simulink model "DDCU_wxt_v02_forA_OpenLoop"  (R2014a)
settings: Solver=FixedStepDiscrete  StartTime=0.0  StopTime=16  FixedStep=0.05  RelTol=1e-3
InitFcn:
  | Veh_Par_wxt
values from neighbouring files (symbols this model uses):
  ag_thr = 0.4*g    (= 3.924)    [Veh_Par_wxt.m]
  B = 2.25    [Veh_Par_wxt.m]
  bra_pre_em = 12    [Veh_Par_wxt.m]
  bra_pre_gz2 = 12/3    (= 4)    [Veh_Par_wxt.m]
  bra_pre_gz34 = 12/3    (= 4)    [Veh_Par_wxt.m]
  bra_pre_yd = 12/2    (= 6)    [Veh_Par_wxt.m]
  brakepre_dem_data = [0 1 2 3 4 5 6 7 8 9 10 11 12]    [Veh_Par_wxt.m]
  brakeTrq_dem_data = [0 218.198 436.396 654.594 872.792 1090.99 1309.188 1527.386 1745.584 1963.782 2181.98 2400.178 2618.376]    [Veh_Par_wxt.m]
  bratrq_max = 4*2618.376    (= 10473.504)    [Veh_Par_wxt.m]
  eff_tran = 0.75    [Veh_Par_wxt.m]
  G = Mass*g    (= 36297)    [Veh_Par_wxt.m]
  kd1 = 1    [Veh_Par_wxt.m]
  kd2 = 1    [Veh_Par_wxt.m]
  kd3 = 1    [Veh_Par_wxt.m]
  ki1 = 1    [Veh_Par_wxt.m]
  ki2 = 1    [Veh_Par_wxt.m]
  ki3 = 1    [Veh_Par_wxt.m]
  kp1 = 1    [Veh_Par_wxt.m]
  kp2 = 1    [Veh_Par_wxt.m]
  kp3 = 1    [Veh_Par_wxt.m]
  L = 3.12    [Veh_Par_wxt.m]
  premax = 12    [Veh_Par_wxt.m]
  Radius = 0.20    (= 0.2)    [Veh_Par_wxt.m]
  s_opt_yi_add = 0.05    [Veh_Par_wxt.m]
  s_opt_zhuan_add = 0.05    [Veh_Par_wxt.m]
  spd_map_mot = [0 100 200 300 360 400 500 600 700 800 900]*tras_ratio    [Veh_Par_wxt.m]
  spdmax = 900*tras_ratio    (= 5580)    [Veh_Par_wxt.m]
  speed_thr_park = 5/3.6/Radius*30/pi    (= 66.3145596216)    [Veh_Par_wxt.m]
  tras_ratio = 6.2    [Veh_Par_wxt.m]
  trq_map_mot = [1200 1200 1200 1200 1200 1080 864 720 617 540 480]/tras_ratio    [Veh_Par_wxt.m]
  trqmax = 80    [Veh_Par_wxt.m]
  v_thr1_b = 5    [Veh_Par_wxt.m]
  v_thr2_b = 20    [Veh_Par_wxt.m]
  v_thr_park = 5    [Veh_Par_wxt.m]
undefined symbols (not defined in the file or in its folder): DiscIntNeverNeededParam, sigbuilder_block
libraries: simulink x169, ec5744lib x9
(part 4 of 13)

== system DDCU_wxt_v02_forA_OpenLoop/OutputSignalProcess/VCU_MCU1_replace/M2Mode ==
  M2Mode : Inport
  Constant{1..4,6..8} (7 alike) : Constant  Value=0  OutDataTypeStr=uint8
  M2ModeRon : Rounding  Operator=round
  M2Mode_1sat : Saturate  UpperLimit=3  LowerLimit=0
  M2Mode_Convert : DataTypeConversion  OutDataTypeStr=uint8
  M2Mode_Convert1 : DataTypeConversion  OutDataTypeStr=uint32
  M2Mode_D : Product  Inputs=*/
  M2Mode_F : Constant  OutDataTypeStr=single
  M2Mode_L : simulink/Logic and Bit Operations/Bitwise Operator  logicop=AND  UseBitMask=on  BitMask=3  BitMaskRealWorld=Stored Integer
  M2Mode_O : Constant  Value=0  OutDataTypeStr=single
  M2Mode_S : ArithShift
  M2Mode_sat : Saturate  UpperLimit=3  LowerLimit=0
  M2Mode_st : Sum  Inputs=+-
  output1 : Outport
  output2 : Outport  Port=2
  output3 : Outport  Port=3
  output4 : Outport  Port=4
  output5 : Outport  Port=5
  output6 : Outport  Port=6
  output7 : Outport  Port=7
  output8 : Outport  Port=8
  wires:
  M2Mode/1 -> M2Mode_sat/1
  M2Mode_sat/1 -> M2Mode_st/1
  M2Mode_O/1 -> M2Mode_st/2
  M2Mode_st/1 -> M2Mode_D/1
  M2Mode_F/1 -> M2Mode_D/2
  M2Mode_D/1 -> M2ModeRon/1
  M2ModeRon/1 -> M2Mode_S/1
  M2Mode_S/1 -> M2Mode_1sat/1
  M2Mode_1sat/1 -> M2Mode_Convert1/1
  M2Mode_Convert1/1 -> M2Mode_L/1
  M2Mode_L/1 -> M2Mode_Convert/1
  M2Mode_Convert/1 -> output5/1
  Constant1/1 -> output1/1
  Constant2/1 -> output2/1
  Constant3/1 -> output3/1
  Constant4/1 -> output4/1
  Constant6/1 -> output6/1
  Constant7/1 -> output7/1
  Constant8/1 -> output8/1

== system DDCU_wxt_v02_forA_OpenLoop/OutputSignalProcess/VCU_MCU1_replace/M2SpeedLimit ==
  M2SpeedLimit : Inport
  Constant{1..6} (6 alike) : Constant  Value=0  OutDataTypeStr=uint8
  M2SpeedLimitBitCov : DataTypeConversion  OutDataTypeStr=uint8
  M2SpeedLimitCOV : DataTypeConversion  OutDataTypeStr=uint8
  M2SpeedLimitRon : Rounding  Operator=round
  M2SpeedLimit_1sat : Saturate  UpperLimit=4095  LowerLimit=0
  M2SpeedLimit_And : simulink/Logic and Bit Operations/Bitwise Operator  logicop=AND  UseBitMask=off  NumInputPorts=2  BitMask=bin2dec('11011001')  BitMaskRealWorld=Stored Integer
  M2SpeedLimit_And_C : Constant  Value=255  OutDataTypeStr=uint32
  M2SpeedLimit_Convert : DataTypeConversion  OutDataTypeStr=uint32
  M2SpeedLimit_D : Product  Inputs=*/
  M2SpeedLimit_D1 : Product  Inputs=*/
  M2SpeedLimit_F : Constant  Value=5  OutDataTypeStr=single
  M2SpeedLimit_L : simulink/Logic and Bit Operations/Bitwise Operator  logicop=AND  UseBitMask=on  BitMask=4095  BitMaskRealWorld=Stored Integer
  M2SpeedLimit_O : Constant  Value=0  OutDataTypeStr=single
  M2SpeedLimit_S : ArithShift
  M2SpeedLimit_sat : Saturate  UpperLimit=20475  LowerLimit=0
  M2SpeedLimit_st : Sum  Inputs=+-
  M2SpeedLimitoutput8_C : Constant  Value=256
  output1 : Outport
  output2 : Outport  Port=2
  output3 : Outport  Port=3
  output4 : Outport  Port=4
  output5 : Outport  Port=5
  output6 : Outport  Port=6
  output7 : Outport  Port=7
  output8 : Outport  Port=8
  wires:
  M2SpeedLimit/1 -> M2SpeedLimit_sat/1
  M2SpeedLimit_sat/1 -> M2SpeedLimit_st/1
  M2SpeedLimit_O/1 -> M2SpeedLimit_st/2
  M2SpeedLimit_st/1 -> M2SpeedLimit_D/1
  M2SpeedLimit_F/1 -> M2SpeedLimit_D/2
  M2SpeedLimit_D/1 -> M2SpeedLimitRon/1
  M2SpeedLimitRon/1 -> M2SpeedLimit_S/1
  M2SpeedLimit_S/1 -> M2SpeedLimit_1sat/1
  M2SpeedLimit_1sat/1 -> M2SpeedLimit_Convert/1
  M2SpeedLimit_Convert/1 -> M2SpeedLimit_L/1
  M2SpeedLimit_L/1 -> M2SpeedLimit_D1/1, M2SpeedLimit_And/1
  M2SpeedLimitoutput8_C/1 -> M2SpeedLimit_D1/2
  M2SpeedLimit_D1/1 -> M2SpeedLimitCOV/1
  M2SpeedLimitCOV/1 -> output8/1
  M2SpeedLimit_And_C/1 -> M2SpeedLimit_And/2
  M2SpeedLimit_And/1 -> M2SpeedLimitBitCov/1
  M2SpeedLimitBitCov/1 -> output7/1
  Constant1/1 -> output1/1
  Constant2/1 -> output2/1
  Constant3/1 -> output3/1
  Constant4/1 -> output4/1
  Constant5/1 -> output5/1
  Constant6/1 -> output6/1

== system DDCU_wxt_v02_forA_OpenLoop/OutputSignalProcess/VCU_MCU1_replace/M2SpeedSet ==
  M2SpeedSet : Inport
  Constant{1..4,7..8} (6 alike) : Constant  Value=0  OutDataTypeStr=uint8
  M2SpeedSetBitCov : DataTypeConversion  OutDataTypeStr=uint8
  M2SpeedSetCOV : DataTypeConversion  OutDataTypeStr=uint8
  M2SpeedSetRon : Rounding  Operator=round
  M2SpeedSet_1sat : Saturate  UpperLimit=65520  LowerLimit=0
  M2SpeedSet_And : simulink/Logic and Bit Operations/Bitwise Operator  logicop=AND  UseBitMask=off  NumInputPorts=2  BitMask=bin2dec('11011001')  BitMaskRealWorld=Stored Integer
  M2SpeedSet_And_C : Constant  Value=255  OutDataTypeStr=uint32
  M2SpeedSet_Convert : DataTypeConversion  OutDataTypeStr=uint32
  M2SpeedSet_D : Product  Inputs=*/
  M2SpeedSet_D1 : Product  Inputs=*/
  M2SpeedSet_F : Constant  Value=5  OutDataTypeStr=single
  M2SpeedSet_L : simulink/Logic and Bit Operations/Bitwise Operator  logicop=AND  UseBitMask=on  BitMask=65520  BitMaskRealWorld=Stored Integer
  M2SpeedSet_O : Constant  Value=-5000  OutDataTypeStr=single
  M2SpeedSet_S : ArithShift  BitShiftNumber=-4
  M2SpeedSet_sat : Saturate  UpperLimit=15475  LowerLimit=-5000
  M2SpeedSet_st : Sum  Inputs=+-
  M2SpeedSetoutput6_C : Constant  Value=256
  output1 : Outport
  output2 : Outport  Port=2
  output3 : Outport  Port=3
  output4 : Outport  Port=4
  output5 : Outport  Port=5
  output6 : Outport  Port=6
  output7 : Outport  Port=7
  output8 : Outport  Port=8
  wires:
  M2SpeedSet/1 -> M2SpeedSet_sat/1
  M2SpeedSet_sat/1 -> M2SpeedSet_st/1
  M2SpeedSet_O/1 -> M2SpeedSet_st/2
  M2SpeedSet_st/1 -> M2SpeedSet_D/1
  M2SpeedSet_F/1 -> M2SpeedSet_D/2
  M2SpeedSet_D/1 -> M2SpeedSetRon/1
  M2SpeedSetRon/1 -> M2SpeedSet_S/1
  M2SpeedSet_S/1 -> M2SpeedSet_1sat/1
  M2SpeedSet_1sat/1 -> M2SpeedSet_Convert/1
  M2SpeedSet_Convert/1 -> M2SpeedSet_L/1
  M2SpeedSet_L/1 -> M2SpeedSet_D1/1, M2SpeedSet_And/1
  M2SpeedSetoutput6_C/1 -> M2SpeedSet_D1/2
  M2SpeedSet_D1/1 -> M2SpeedSetCOV/1
  M2SpeedSetCOV/1 -> output6/1
  M2SpeedSet_And_C/1 -> M2SpeedSet_And/2
  M2SpeedSet_And/1 -> M2SpeedSetBitCov/1
  M2SpeedSetBitCov/1 -> output5/1
  Constant1/1 -> output1/1
  Constant2/1 -> output2/1
  Constant3/1 -> output3/1
  Constant4/1 -> output4/1
  Constant7/1 -> output7/1
  Constant8/1 -> output8/1

== system DDCU_wxt_v02_forA_OpenLoop/OutputSignalProcess/VCU_MCU1_replace/MCU1HeartBeat ==
  MCU1HeartBeat : Inport
  Constant{1..7} (7 alike) : Constant  Value=0  OutDataTypeStr=uint8
  MCU1HeartBeatRon : Rounding  Operator=round
  MCU1HeartBeat_1sat : Saturate  UpperLimit=240  LowerLimit=0
  MCU1HeartBeat_Convert : DataTypeConversion  OutDataTypeStr=uint8
  MCU1HeartBeat_Convert1 : DataTypeConversion  OutDataTypeStr=uint32
  MCU1HeartBeat_D : Product  Inputs=*/
  MCU1HeartBeat_F : Constant  OutDataTypeStr=single
  MCU1HeartBeat_L : simulink/Logic and Bit Operations/Bitwise Operator  logicop=AND  UseBitMask=on  BitMask=240  BitMaskRealWorld=Stored Integer
  MCU1HeartBeat_O : Constant  Value=0  OutDataTypeStr=single
  MCU1HeartBeat_S : ArithShift  BitShiftNumber=-4
  MCU1HeartBeat_sat : Saturate  UpperLimit=15  LowerLimit=0
  MCU1HeartBeat_st : Sum  Inputs=+-
  output1 : Outport
  output2 : Outport  Port=2
  output3 : Outport  Port=3
  output4 : Outport  Port=4
  output5 : Outport  Port=5
  output6 : Outport  Port=6
  output7 : Outport  Port=7
  output8 : Outport  Port=8
  wires:
  MCU1HeartBeat/1 -> MCU1HeartBeat_sat/1
  MCU1HeartBeat_sat/1 -> MCU1HeartBeat_st/1
  MCU1HeartBeat_O/1 -> MCU1HeartBeat_st/2
  MCU1HeartBeat_st/1 -> MCU1HeartBeat_D/1
  MCU1HeartBeat_F/1 -> MCU1HeartBeat_D/2
  MCU1HeartBeat_D/1 -> MCU1HeartBeatRon/1
  MCU1HeartBeatRon/1 -> MCU1HeartBeat_S/1
  MCU1HeartBeat_S/1 -> MCU1HeartBeat_1sat/1
  MCU1HeartBeat_1sat/1 -> MCU1HeartBeat_Convert1/1
  MCU1HeartBeat_Convert1/1 -> MCU1HeartBeat_L/1
  MCU1HeartBeat_L/1 -> MCU1HeartBeat_Convert/1
  MCU1HeartBeat_Convert/1 -> output8/1
  Constant1/1 -> output1/1
  Constant2/1 -> output2/1
  Constant3/1 -> output3/1
  Constant4/1 -> output4/1
  Constant5/1 -> output5/1
  Constant6/1 -> output6/1
  Constant7/1 -> output7/1

== system DDCU_wxt_v02_forA_OpenLoop/OutputSignalProcess/VCU_MCU2/M3Drive ==
  M3Drive : Inport
  Constant{2..8} (7 alike) : Constant  Value=0  OutDataTypeStr=uint8
  M3DriveRon : Rounding  Operator=round
  M3Drive_1sat : Saturate  UpperLimit=48  LowerLimit=0
  M3Drive_Convert : DataTypeConversion  OutDataTypeStr=uint8
  M3Drive_Convert1 : DataTypeConversion  OutDataTypeStr=uint32
  M3Drive_D : Product  Inputs=*/
  M3Drive_F : Constant  OutDataTypeStr=single
  M3Drive_L : simulink/Logic and Bit Operations/Bitwise Operator  logicop=AND  UseBitMask=on  BitMask=48  BitMaskRealWorld=Stored Integer
  M3Drive_O : Constant  Value=0  OutDataTypeStr=single
  M3Drive_S : ArithShift  BitShiftNumber=-4
  M3Drive_sat : Saturate  UpperLimit=3  LowerLimit=0
  M3Drive_st : Sum  Inputs=+-
  output1 : Outport
  output2 : Outport  Port=2
  output3 : Outport  Port=3
  output4 : Outport  Port=4
  output5 : Outport  Port=5
  output6 : Outport  Port=6
  output7 : Outport  Port=7
  output8 : Outport  Port=8
  wires:
  M3Drive/1 -> M3Drive_sat/1
  M3Drive_sat/1 -> M3Drive_st/1
  M3Drive_O/1 -> M3Drive_st/2
  M3Drive_st/1 -> M3Drive_D/1
  M3Drive_F/1 -> M3Drive_D/2
  M3Drive_D/1 -> M3DriveRon/1
  M3DriveRon/1 -> M3Drive_S/1
  M3Drive_S/1 -> M3Drive_1sat/1
  M3Drive_1sat/1 -> M3Drive_Convert1/1
  M3Drive_Convert1/1 -> M3Drive_L/1
  M3Drive_L/1 -> M3Drive_Convert/1
  M3Drive_Convert/1 -> output1/1
  Constant2/1 -> output2/1
  Constant3/1 -> output3/1
  Constant4/1 -> output4/1
  Constant5/1 -> output5/1
  Constant6/1 -> output6/1
  Constant7/1 -> output7/1
  Constant8/1 -> output8/1

== system DDCU_wxt_v02_forA_OpenLoop/OutputSignalProcess/VCU_MCU2/M3Enable ==
  M3Enable : Inport
  Constant{2..8} (7 alike) : Constant  Value=0  OutDataTypeStr=uint8
  M3EnableRon : Rounding  Operator=round
  M3Enable_1sat : Saturate  UpperLimit=3  LowerLimit=0
  M3Enable_Convert : DataTypeConversion  OutDataTypeStr=uint8
  M3Enable_Convert1 : DataTypeConversion  OutDataTypeStr=uint32
  M3Enable_D : Product  Inputs=*/
  M3Enable_F : Constant  OutDataTypeStr=single
  M3Enable_L : simulink/Logic and Bit Operations/Bitwise Operator  logicop=AND  UseBitMask=on  BitMask=3  BitMaskRealWorld=Stored Integer
  M3Enable_O : Constant  Value=0  OutDataTypeStr=single
  M3Enable_S : ArithShift
  M3Enable_sat : Saturate  UpperLimit=3  LowerLimit=0
  M3Enable_st : Sum  Inputs=+-
  output1 : Outport
  output2 : Outport  Port=2
  output3 : Outport  Port=3
  output4 : Outport  Port=4
  output5 : Outport  Port=5
  output6 : Outport  Port=6
  output7 : Outport  Port=7
  output8 : Outport  Port=8
  wires:
  M3Enable/1 -> M3Enable_sat/1
  M3Enable_sat/1 -> M3Enable_st/1
  M3Enable_O/1 -> M3Enable_st/2
  M3Enable_st/1 -> M3Enable_D/1
  M3Enable_F/1 -> M3Enable_D/2
  M3Enable_D/1 -> M3EnableRon/1
  M3EnableRon/1 -> M3Enable_S/1
  M3Enable_S/1 -> M3Enable_1sat/1
  M3Enable_1sat/1 -> M3Enable_Convert1/1
  M3Enable_Convert1/1 -> M3Enable_L/1
  M3Enable_L/1 -> M3Enable_Convert/1
  M3Enable_Convert/1 -> output1/1
  Constant2/1 -> output2/1
  Constant3/1 -> output3/1
  Constant4/1 -> output4/1
  Constant5/1 -> output5/1
  Constant6/1 -> output6/1
  Constant7/1 -> output7/1
  Constant8/1 -> output8/1

== system DDCU_wxt_v02_forA_OpenLoop/OutputSignalProcess/VCU_MCU2/M3Mode ==
  M3Mode : Inport
  Constant{2..8} (7 alike) : Constant  Value=0  OutDataTypeStr=uint8
  M3ModeRon : Rounding  Operator=round
  M3Mode_1sat : Saturate  UpperLimit=12  LowerLimit=0
  M3Mode_Convert : DataTypeConversion  OutDataTypeStr=uint8
  M3Mode_Convert1 : DataTypeConversion  OutDataTypeStr=uint32
  M3Mode_D : Product  Inputs=*/
  M3Mode_F : Constant  OutDataTypeStr=single
  M3Mode_L : simulink/Logic and Bit Operations/Bitwise Operator  logicop=AND  UseBitMask=on  BitMask=12  BitMaskRealWorld=Stored Integer
  M3Mode_O : Constant  Value=0  OutDataTypeStr=single
  M3Mode_S : ArithShift  BitShiftNumber=-2
  M3Mode_sat : Saturate  UpperLimit=3  LowerLimit=0
  M3Mode_st : Sum  Inputs=+-
  output1 : Outport
  output2 : Outport  Port=2
  output3 : Outport  Port=3
  output4 : Outport  Port=4
  output5 : Outport  Port=5
  output6 : Outport  Port=6
  output7 : Outport  Port=7
  output8 : Outport  Port=8
  wires:
  M3Mode/1 -> M3Mode_sat/1
  M3Mode_sat/1 -> M3Mode_st/1
  M3Mode_O/1 -> M3Mode_st/2
  M3Mode_st/1 -> M3Mode_D/1
  M3Mode_F/1 -> M3Mode_D/2
  M3Mode_D/1 -> M3ModeRon/1
  M3ModeRon/1 -> M3Mode_S/1
  M3Mode_S/1 -> M3Mode_1sat/1
  M3Mode_1sat/1 -> M3Mode_Convert1/1
  M3Mode_Convert1/1 -> M3Mode_L/1
  M3Mode_L/1 -> M3Mode_Convert/1
  M3Mode_Convert/1 -> output1/1
  Constant2/1 -> output2/1
  Constant3/1 -> output3/1
  Constant4/1 -> output4/1
  Constant5/1 -> output5/1
  Constant6/1 -> output6/1
  Constant7/1 -> output7/1
  Constant8/1 -> output8/1

== system DDCU_wxt_v02_forA_OpenLoop/OutputSignalProcess/VCU_MCU2/M3SpeedLimit ==
  M3SpeedLimit : Inport
  BitCov : DataTypeConversion  OutDataTypeStr=uint8
  Constant{1..2,5..8} (6 alike) : Constant  Value=0  OutDataTypeStr=uint8
  M3SpeedLimitCOV : DataTypeConversion  OutDataTypeStr=uint8
  M3SpeedLimitRon : Rounding  Operator=round
  M3SpeedLimit_1sat : Saturate  UpperLimit=16380  LowerLimit=0
  M3SpeedLimit_And : simulink/Logic and Bit Operations/Bitwise Operator  logicop=AND  UseBitMask=off  NumInputPorts=2  BitMask=bin2dec('11011001')  BitMaskRealWorld=Stored Integer
  M3SpeedLimit_And_C : Constant  Value=255  OutDataTypeStr=uint32
  M3SpeedLimit_Convert : DataTypeConversion  OutDataTypeStr=uint32
  M3SpeedLimit_D : Product  Inputs=*/
  M3SpeedLimit_D1 : Product  Inputs=*/
  M3SpeedLimit_F : Constant  Value=5  OutDataTypeStr=single
  M3SpeedLimit_L : simulink/Logic and Bit Operations/Bitwise Operator  logicop=AND  UseBitMask=on  BitMask=16380  BitMaskRealWorld=Stored Integer
  M3SpeedLimit_O : Constant  Value=0  OutDataTypeStr=single
  M3SpeedLimit_S : ArithShift  BitShiftNumber=-2
  M3SpeedLimit_sat : Saturate  UpperLimit=20475  LowerLimit=0
  M3SpeedLimit_st : Sum  Inputs=+-
  M3SpeedLimitoutput4_C : Constant  Value=256
  output1 : Outport
  output2 : Outport  Port=2
  output3 : Outport  Port=3
  output4 : Outport  Port=4
  output5 : Outport  Port=5
  output6 : Outport  Port=6
  output7 : Outport  Port=7
  output8 : Outport  Port=8
  wires:
  M3SpeedLimit/1 -> M3SpeedLimit_sat/1
  M3SpeedLimit_sat/1 -> M3SpeedLimit_st/1
  M3SpeedLimit_O/1 -> M3SpeedLimit_st/2
  M3SpeedLimit_st/1 -> M3SpeedLimit_D/1
  M3SpeedLimit_F/1 -> M3SpeedLimit_D/2
  M3SpeedLimit_D/1 -> M3SpeedLimitRon/1
  M3SpeedLimitRon/1 -> M3SpeedLimit_S/1
  M3SpeedLimit_S/1 -> M3SpeedLimit_1sat/1
  M3SpeedLimit_1sat/1 -> M3SpeedLimit_Convert/1
  M3SpeedLimit_Convert/1 -> M3SpeedLimit_L/1
  M3SpeedLimit_L/1 -> M3SpeedLimit_D1/1, M3SpeedLimit_And/1
  M3SpeedLimitoutput4_C/1 -> M3SpeedLimit_D1/2
  M3SpeedLimit_D1/1 -> M3SpeedLimitCOV/1
  M3SpeedLimitCOV/1 -> output4/1
  M3SpeedLimit_And_C/1 -> M3SpeedLimit_And/2
  M3SpeedLimit_And/1 -> BitCov/1
  BitCov/1 -> output3/1
  Constant1/1 -> output1/1
  Constant2/1 -> output2/1
  Constant5/1 -> output5/1
  Constant6/1 -> output6/1
  Constant7/1 -> output7/1
  Constant8/1 -> output8/1

== system DDCU_wxt_v02_forA_OpenLoop/OutputSignalProcess/VCU_MCU2/M3TorqueSet ==
  M3TorqueSet : Inport
  Constant{4..8} (5 alike) : Constant  Value=0  OutDataTypeStr=uint8
  M3TorqueSetBitCov : DataTypeConversion  OutDataTypeStr=uint32
  M3TorqueSetBitCov1 : DataTypeConversion  OutDataTypeStr=uint8
  M3TorqueSetCOV : DataTypeConversion  OutDataTypeStr=uint8
  M3TorqueSetCOV1 : DataTypeConversion  OutDataTypeStr=uint8
  M3TorqueSetRon : Rounding  Operator=round
  M3TorqueSet_1sat : Saturate  UpperLimit=262080  LowerLimit=0
  M3TorqueSet_And : simulink/Logic and Bit Operations/Bitwise Operator  logicop=AND  UseBitMask=off  NumInputPorts=2  BitMask=bin2dec('11011001')  BitMaskRealWorld=Stored Integer
  M3TorqueSet_And1 : simulink/Logic and Bit Operations/Bitwise Operator  logicop=AND  UseBitMask=off  NumInputPorts=2  BitMask=bin2dec('11011001')  BitMaskRealWorld=Stored Integer
  M3TorqueSet_And1_C : Constant  Value=255  OutDataTypeStr=uint32
  M3TorqueSet_And_C : Constant  Value=65535
  M3TorqueSet_Convert : DataTypeConversion  OutDataTypeStr=uint32
  M3TorqueSet_D : Product  Inputs=*/
  M3TorqueSet_D1 : Product  Inputs=*/
  M3TorqueSet_D2 : Product  Inputs=*/
  M3TorqueSet_F : Constant  Value=0.25  OutDataTypeStr=single
  M3TorqueSet_L : simulink/Logic and Bit Operations/Bitwise Operator  logicop=AND  UseBitMask=on  BitMask=262080  BitMaskRealWorld=Stored Integer
  M3TorqueSet_O : Constant  Value=-300  OutDataTypeStr=single
  M3TorqueSet_S : ArithShift  BitShiftNumber=-6
  M3TorqueSet_sat : Saturate  UpperLimit=723.75  LowerLimit=-300
  M3TorqueSet_st : Sum  Inputs=+-
  M3TorqueSetoutput2_C : Constant  Value=256
  M3TorqueSetoutput3_C : Constant  Value=65536
  output1 : Outport
  output2 : Outport  Port=2
  output3 : Outport  Port=3
  output4 : Outport  Port=4
  output5 : Outport  Port=5
  output6 : Outport  Port=6
  output7 : Outport  Port=7
  output8 : Outport  Port=8
  wires:
  M3TorqueSet/1 -> M3TorqueSet_sat/1
  M3TorqueSet_sat/1 -> M3TorqueSet_st/1
  M3TorqueSet_O/1 -> M3TorqueSet_st/2
  M3TorqueSet_st/1 -> M3TorqueSet_D/1
  M3TorqueSet_F/1 -> M3TorqueSet_D/2
  M3TorqueSet_D/1 -> M3TorqueSetRon/1
  M3TorqueSetRon/1 -> M3TorqueSet_S/1
  M3TorqueSet_S/1 -> M3TorqueSet_1sat/1
  M3TorqueSet_1sat/1 -> M3TorqueSet_Convert/1
  M3TorqueSet_Convert/1 -> M3TorqueSet_L/1
  M3TorqueSet_L/1 -> M3TorqueSet_D1/1, M3TorqueSet_And/1, M3TorqueSet_And1/1
  M3TorqueSetoutput3_C/1 -> M3TorqueSet_D1/2
  M3TorqueSet_D1/1 -> M3TorqueSetCOV/1
  M3TorqueSetCOV/1 -> output3/1
  M3TorqueSet_And_C/1 -> M3TorqueSetBitCov/1
  M3TorqueSetBitCov/1 -> M3TorqueSet_And/2
  M3TorqueSet_And/1 -> M3TorqueSet_D2/1
  M3TorqueSetoutput2_C/1 -> M3TorqueSet_D2/2
  M3TorqueSet_D2/1 -> M3TorqueSetCOV1/1
  M3TorqueSetCOV1/1 -> output2/1
  M3TorqueSet_And1_C/1 -> M3TorqueSet_And1/2
  M3TorqueSet_And1/1 -> M3TorqueSetBitCov1/1
  M3TorqueSetBitCov1/1 -> output1/1
  Constant4/1 -> output4/1
  Constant5/1 -> output5/1
  Constant6/1 -> output6/1
  Constant7/1 -> output7/1
  Constant8/1 -> output8/1

== system DDCU_wxt_v02_forA_OpenLoop/OutputSignalProcess/VCU_MCU2/M4Drive ==
  M4Drive : Inport
  Constant{1..4,6..8} (7 alike) : Constant  Value=0  OutDataTypeStr=uint8
  M4DriveRon : Rounding  Operator=round
  M4Drive_1sat : Saturate  UpperLimit=12  LowerLimit=0
  M4Drive_Convert : DataTypeConversion  OutDataTypeStr=uint8
  M4Drive_Convert1 : DataTypeConversion  OutDataTypeStr=uint32
  M4Drive_D : Product  Inputs=*/
  M4Drive_F : Constant  OutDataTypeStr=single
  M4Drive_L : simulink/Logic and Bit Operations/Bitwise Operator  logicop=AND  UseBitMask=on  BitMask=12  BitMaskRealWorld=Stored Integer
  M4Drive_O : Constant  Value=0  OutDataTypeStr=single
  M4Drive_S : ArithShift  BitShiftNumber=-2
  M4Drive_sat : Saturate  UpperLimit=3  LowerLimit=0
  M4Drive_st : Sum  Inputs=+-
  output1 : Outport
  output2 : Outport  Port=2
  output3 : Outport  Port=3
  output4 : Outport  Port=4
  output5 : Outport  Port=5
  output6 : Outport  Port=6
  output7 : Outport  Port=7
  output8 : Outport  Port=8
  wires:
  M4Drive/1 -> M4Drive_sat/1
  M4Drive_sat/1 -> M4Drive_st/1
  M4Drive_O/1 -> M4Drive_st/2
  M4Drive_st/1 -> M4Drive_D/1
  M4Drive_F/1 -> M4Drive_D/2
  M4Drive_D/1 -> M4DriveRon/1
  M4DriveRon/1 -> M4Drive_S/1
  M4Drive_S/1 -> M4Drive_1sat/1
  M4Drive_1sat/1 -> M4Drive_Convert1/1
  M4Drive_Convert1/1 -> M4Drive_L/1
  M4Drive_L/1 -> M4Drive_Convert/1
  M4Drive_Convert/1 -> output5/1
  Constant1/1 -> output1/1
  Constant2/1 -> output2/1
  Constant3/1 -> output3/1
  Constant4/1 -> output4/1
  Constant6/1 -> output6/1
  Constant7/1 -> output7/1
  Constant8/1 -> output8/1

== matlab function DDCU_wxt_v02_forA_OpenLoop/MainControl/mode_control/center_steer/center_steer/容错控制/MATLAB Function ==
  data: trq_dem_l input; trq_dem_lf output; trq_dem_r input; trqlim_lf input; trqlim_lr input; trqlim_rf input; trqlim_rr input; guzhang_lf input; guzhang_lr input; guzhang_rf input; guzhang_rr input; trq_dem_lr output; trq_dem_rf output; trq_dem_rr output; bra_pre_l output; bra_pre_r output; bra_pre_yd input; mode output
function [trq_dem_lf,trq_dem_lr,trq_dem_rf,trq_dem_rr,bra_pre_l,bra_pre_r,mode] = fcn(trq_dem_l,trq_dem_r,trqlim_lf,trqlim_lr,trqlim_rf,trqlim_rr,guzhang_lf,guzhang_lr,guzhang_rf,guzhang_rr,bra_pre_yd)
%#codegen
if guzhang_lf==0 && guzhang_lr==0 && guzhang_rf==0 && guzhang_rr==0    %0电机故障,平均分配
    trq_dem_lf=trq_dem_l/2;
    trq_dem_lr=trq_dem_l/2;
    trq_dem_rf=trq_dem_r/2;
    trq_dem_rr=trq_dem_r/2;
    bra_pre_l=0;
    bra_pre_r=0;
    mode=1;
elseif  guzhang_lf==1 && guzhang_lr==0 && guzhang_rf==0 && guzhang_rr==0  %1电机故障，同侧电机进行力矩转移,跟行车不同，对侧不降扭。
    trq_dem_lf=0;
    trq_dem_lr=min(trq_dem_l,trqlim_lr);
    trq_dem_rf=trq_dem_r/2;
    trq_dem_rr=trq_dem_r/2;
    bra_pre_l=0;
    bra_pre_r=0;
    mode=2;
elseif  guzhang_lf==0 && guzhang_lr==1 && guzhang_rf==0 && guzhang_rr==0
    trq_dem_lf=min(trq_dem_l,trqlim_lf);
    trq_dem_lr=0;
    trq_dem_rf=trq_dem_r/2;
    trq_dem_rr=trq_dem_r/2;
    bra_pre_l=0;
    bra_pre_r=0;
    mode=3;
elseif  guzhang_lf==0 && guzhang_lr==0 && guzhang_rf==1 && guzhang_rr==0
    trq_dem_rf=0;
    trq_dem_rr=min(trq_dem_r,trqlim_rr);
    trq_dem_lf=trq_dem_l/2;
    trq_dem_lr=trq_dem_l/2;
    bra_pre_l=0;
    bra_pre_r=0;
    mode=4;
elseif  guzhang_lf==0 && guzhang_lr==0 && guzhang_rf==0 && guzhang_rr==1
    trq_dem_rf=min(trq_dem_r,trqlim_rf);
    trq_dem_rr=0;
    trq_dem_lf=trq_dem_l/2;
    trq_dem_lr=trq_dem_l/2;
    bra_pre_l=0;
    bra_pre_r=0;
    mode=5;
elseif  guzhang_lf==1 && guzhang_lr==1 && guzhang_rf==0 && guzhang_rr==0  %2电机故障，左侧双电机故障，左侧履带施加制动，改为原地转向
    trq_dem_lf=0;
    trq_dem_lr=0;
    trq_dem_rf=trq_dem_r/2;
    trq_dem_rr=trq_dem_r/2;
    bra_pre_l=bra_pre_yd;
    bra_pre_r=0;
    mode=6;
elseif  guzhang_lf==0 && guzhang_lr==0 && guzhang_rf==1 && guzhang_rr==1  %右侧双电机故障
    trq_dem_lf=trq_dem_l/2;
    trq_dem_lr=trq_dem_l/2;
    trq_dem_rf=0;
    trq_dem_rr=0;
    bra_pre_l=0;
    bra_pre_r=bra_pre_yd;
    mode=7;
elseif  guzhang_lf==1 && guzhang_lr==0 && guzhang_rf==1 && guzhang_rr==0 %2电机故障，对侧双电机故障,有4种情况,前两电机故障
    trq_dem_lf=0;
    trq_dem_rf=0;
    trq_dem_lr=min(trq_dem_l,trqlim_lr);
    trq_dem_rr=min(trq_dem_r,trqlim_rr);
    bra_pre_l=0;
    bra_pre_r=0;
    mode=8;
elseif  guzhang_lf==0 && guzhang_lr==1 && guzhang_rf==0 && guzhang_rr==1 %后两电机故障
    trq_dem_lr=0;
    trq_dem_rr=0;
    trq_dem_lf=min(trq_dem_l,trqlim_lf);
    trq_dem_rf=min(trq_dem_r,trqlim_rf);
    bra_pre_l=0;
    bra_pre_r=0;
    mode=9;
elseif  guzhang_lf==1 && guzhang_lr==0 && guzhang_rf==0 && guzhang_rr==1 %左前电机和右后电机故障
    trq_dem_lf=0;
    trq_dem_rr=0;
    trq_dem_lr=min(trq_dem_l,trqlim_lr);
    trq_dem_rf=min(trq_dem_r,trqlim_rf);
    bra_pre_l=0;
    bra_pre_r=0;
    mode=10;
elseif  guzhang_lf==0 && guzhang_lr==1 && guzhang_rf==1 && guzhang_rr==0 %左后电机和右前电机故障
    trq_dem_lr=0;
    trq_dem_rf=0;
    trq_dem_lf=min(trq_dem_l,trqlim_lf);
    trq_dem_rr=min(trq_dem_r,trqlim_rr);
    bra_pre_l=0;
    bra_pre_r=0;
    mode=11;
elseif guzhang_lf==1 && guzhang_lr==1 && guzhang_rf==1 && guzhang_rr==0   % 三电机故障
    trq_dem_lf=0;
    trq_dem_lr=0;
    trq_dem_rf=0;
    trq_dem_rr=min(trq_dem_r,trqlim_rr);
    bra_pre_l=bra_pre_yd;
    bra_pre_r=0;
    mode=12;
elseif guzhang_lf==1 && guzhang_lr==1 && guzhang_rf==0 && guzhang_rr==1
    trq_dem_lf=0;
    trq_dem_lr=0;
    trq_dem_rf=min(trq_dem_r,trqlim_rf);
    trq_dem_rr=0;
    bra_pre_l=bra_pre_yd;
    bra_pre_r=0;
    mode=13;
elseif guzhang_lf==1 && guzhang_lr==0 && guzhang_rf==1 && guzhang_rr==1
    trq_dem_lf=0;
    trq_dem_lr=min(trq_dem_l,trqlim_lr);
    trq_dem_rf=0;
    trq_dem_rr=0;
    bra_pre_l=0;
    bra_pre_r=bra_pre_yd;
    mode=14;
elseif guzhang_lf==0 && guzhang_lr==1 && guzhang_rf==1 && guzhang_rr==1
    trq_dem_lf=min(trq_dem_l,trqlim_lf);
    trq_dem_lr=0;
    trq_dem_rf=0;
    trq_dem_rr=0;
    bra_pre_l=0;
    bra_pre_r=bra_pre_yd;
    mode=15;
else
    %     guzhang_lf==1 && guzhang_lr==1 && guzhang_rf==1 && guzhang_rr==1 %四电机故障
    trq_dem_lf=0;
    trq_dem_lr=0;
    trq_dem_rf=0;
    trq_dem_rr=0;
    bra_pre_l=0;
    bra_pre_r=0;
    mode=16;
end
trq_dem_lf=min(trqlim_lf,trq_dem_lf);trq_dem_lf=max(0,trq_dem_lf);
trq_dem_lr=min(trqlim_lr,trq_dem_lr);trq_dem_lr=max(0,trq_dem_lr);
trq_dem_rf=min(trqlim_rf,trq_dem_rf);trq_dem_rf=max(0,trq_dem_rf);
trq_dem_rr=min(trqlim_rr,trq_dem_rr);trq_dem_rr=max(0,trq_dem_rr);
bra_pre_l=bra_pre_l;
bra_pre_r=bra_pre_r;
end

== system DDCU_wxt_v02_forA_OpenLoop/OutputSignalProcess/VCU_MCU2/M4Enable ==
  M4Enable : Inport
  Constant{1..3,5..8} (7 alike) : Constant  Value=0  OutDataTypeStr=uint8
  M4EnableRon : Rounding  Operator=round
  M4Enable_1sat : Saturate  UpperLimit=192  LowerLimit=0
  M4Enable_Convert : DataTypeConversion  OutDataTypeStr=uint8
  M4Enable_Convert1 : DataTypeConversion  OutDataTypeStr=uint32
  M4Enable_D : Product  Inputs=*/
  M4Enable_F : Constant  OutDataTypeStr=single
  M4Enable_L : simulink/Logic and Bit Operations/Bitwise Operator  logicop=AND  UseBitMask=on  BitMask=192  BitMaskRealWorld=Stored Integer
  M4Enable_O : Constant  Value=0  OutDataTypeStr=single
  M4Enable_S : ArithShift  BitShiftNumber=-6
  M4Enable_sat : Saturate  UpperLimit=3  LowerLimit=0
  M4Enable_st : Sum  Inputs=+-
  output1 : Outport
  output2 : Outport  Port=2
  output3 : Outport  Port=3
  output4 : Outport  Port=4
  output5 : Outport  Port=5
  output6 : Outport  Port=6
  output7 : Outport  Port=7
  output8 : Outport  Port=8
  wires:
  M4Enable/1 -> M4Enable_sat/1
  M4Enable_sat/1 -> M4Enable_st/1
  M4Enable_O/1 -> M4Enable_st/2
  M4Enable_st/1 -> M4Enable_D/1
  M4Enable_F/1 -> M4Enable_D/2
  M4Enable_D/1 -> M4EnableRon/1
  M4EnableRon/1 -> M4Enable_S/1
  M4Enable_S/1 -> M4Enable_1sat/1
  M4Enable_1sat/1 -> M4Enable_Convert1/1
  M4Enable_Convert1/1 -> M4Enable_L/1
  M4Enable_L/1 -> M4Enable_Convert/1
  M4Enable_Convert/1 -> output4/1
  Constant1/1 -> output1/1
  Constant2/1 -> output2/1
  Constant3/1 -> output3/1
  Constant5/1 -> output5/1
  Constant6/1 -> output6/1
  Constant7/1 -> output7/1
  Constant8/1 -> output8/1

== system DDCU_wxt_v02_forA_OpenLoop/OutputSignalProcess/VCU_MCU2/M4Mode ==
  M4Mode : Inport
  Constant{1..4,6..8} (7 alike) : Constant  Value=0  OutDataTypeStr=uint8
  M4ModeRon : Rounding  Operator=round
  M4Mode_1sat : Saturate  UpperLimit=3  LowerLimit=0
  M4Mode_Convert : DataTypeConversion  OutDataTypeStr=uint8
  M4Mode_Convert1 : DataTypeConversion  OutDataTypeStr=uint32
  M4Mode_D : Product  Inputs=*/
  M4Mode_F : Constant  OutDataTypeStr=single
  M4Mode_L : simulink/Logic and Bit Operations/Bitwise Operator  logicop=AND  UseBitMask=on  BitMask=3  BitMaskRealWorld=Stored Integer
  M4Mode_O : Constant  Value=0  OutDataTypeStr=single
  M4Mode_S : ArithShift
  M4Mode_sat : Saturate  UpperLimit=3  LowerLimit=0
  M4Mode_st : Sum  Inputs=+-
  output1 : Outport
  output2 : Outport  Port=2
  output3 : Outport  Port=3
  output4 : Outport  Port=4
  output5 : Outport  Port=5
  output6 : Outport  Port=6
  output7 : Outport  Port=7
  output8 : Outport  Port=8
  wires:
  M4Mode/1 -> M4Mode_sat/1
  M4Mode_sat/1 -> M4Mode_st/1
  M4Mode_O/1 -> M4Mode_st/2
  M4Mode_st/1 -> M4Mode_D/1
  M4Mode_F/1 -> M4Mode_D/2
  M4Mode_D/1 -> M4ModeRon/1
  M4ModeRon/1 -> M4Mode_S/1
  M4Mode_S/1 -> M4Mode_1sat/1
  M4Mode_1sat/1 -> M4Mode_Convert1/1
  M4Mode_Convert1/1 -> M4Mode_L/1
  M4Mode_L/1 -> M4Mode_Convert/1
  M4Mode_Convert/1 -> output5/1
  Constant1/1 -> output1/1
  Constant2/1 -> output2/1
  Constant3/1 -> output3/1
  Constant4/1 -> output4/1
  Constant6/1 -> output6/1
  Constant7/1 -> output7/1
  Constant8/1 -> output8/1

== system DDCU_wxt_v02_forA_OpenLoop/OutputSignalProcess/VCU_MCU2/M4SpeedLimit ==
  M4SpeedLimit : Inport
  Constant{1..6} (6 alike) : Constant  Value=0  OutDataTypeStr=uint8
  M4SpeedLimitBitCov : DataTypeConversion  OutDataTypeStr=uint8
  M4SpeedLimitCOV : DataTypeConversion  OutDataTypeStr=uint8
  M4SpeedLimitRon : Rounding  Operator=round
  M4SpeedLimit_1sat : Saturate  UpperLimit=4095  LowerLimit=0
  M4SpeedLimit_And : simulink/Logic and Bit Operations/Bitwise Operator  logicop=AND  UseBitMask=off  NumInputPorts=2  BitMask=bin2dec('11011001')  BitMaskRealWorld=Stored Integer
  M4SpeedLimit_And_C : Constant  Value=255  OutDataTypeStr=uint32
  M4SpeedLimit_Convert : DataTypeConversion  OutDataTypeStr=uint32
  M4SpeedLimit_D : Product  Inputs=*/
  M4SpeedLimit_D1 : Product  Inputs=*/
  M4SpeedLimit_F : Constant  Value=5  OutDataTypeStr=single
  M4SpeedLimit_L : simulink/Logic and Bit Operations/Bitwise Operator  logicop=AND  UseBitMask=on  BitMask=4095  BitMaskRealWorld=Stored Integer
  M4SpeedLimit_O : Constant  Value=0  OutDataTypeStr=single
  M4SpeedLimit_S : ArithShift
  M4SpeedLimit_sat : Saturate  UpperLimit=20475  LowerLimit=0
  M4SpeedLimit_st : Sum  Inputs=+-
  M4SpeedLimitoutput8_C : Constant  Value=256
  output1 : Outport
  output2 : Outport  Port=2
  output3 : Outport  Port=3
  output4 : Outport  Port=4
  output5 : Outport  Port=5
  output6 : Outport  Port=6
  output7 : Outport  Port=7
  output8 : Outport  Port=8
  wires:
  M4SpeedLimit/1 -> M4SpeedLimit_sat/1
  M4SpeedLimit_sat/1 -> M4SpeedLimit_st/1
  M4SpeedLimit_O/1 -> M4SpeedLimit_st/2
  M4SpeedLimit_st/1 -> M4SpeedLimit_D/1
  M4SpeedLimit_F/1 -> M4SpeedLimit_D/2
  M4SpeedLimit_D/1 -> M4SpeedLimitRon/1
  M4SpeedLimitRon/1 -> M4SpeedLimit_S/1
  M4SpeedLimit_S/1 -> M4SpeedLimit_1sat/1
  M4SpeedLimit_1sat/1 -> M4SpeedLimit_Convert/1
  M4SpeedLimit_Convert/1 -> M4SpeedLimit_L/1
  M4SpeedLimit_L/1 -> M4SpeedLimit_D1/1, M4SpeedLimit_And/1
  M4SpeedLimitoutput8_C/1 -> M4SpeedLimit_D1/2
  M4SpeedLimit_D1/1 -> M4SpeedLimitCOV/1
  M4SpeedLimitCOV/1 -> output8/1
  M4SpeedLimit_And_C/1 -> M4SpeedLimit_And/2
  M4SpeedLimit_And/1 -> M4SpeedLimitBitCov/1
  M4SpeedLimitBitCov/1 -> output7/1
  Constant1/1 -> output1/1
  Constant2/1 -> output2/1
  Constant3/1 -> output3/1
  Constant4/1 -> output4/1
  Constant5/1 -> output5/1
  Constant6/1 -> output6/1

== system DDCU_wxt_v02_forA_OpenLoop/OutputSignalProcess/VCU_MCU2/M4TorqueSet ==
  M4TorqueSet : Inport
  Constant{1..4,7..8} (6 alike) : Constant  Value=0  OutDataTypeStr=uint8
  M4TorqueSetBitCov : DataTypeConversion  OutDataTypeStr=uint8
  M4TorqueSetCOV : DataTypeConversion  OutDataTypeStr=uint8
  M4TorqueSetRon : Rounding  Operator=round
  M4TorqueSet_1sat : Saturate  UpperLimit=65520  LowerLimit=0
  M4TorqueSet_And : simulink/Logic and Bit Operations/Bitwise Operator  logicop=AND  UseBitMask=off  NumInputPorts=2  BitMask=bin2dec('11011001')  BitMaskRealWorld=Stored Integer
  M4TorqueSet_And_C : Constant  Value=255  OutDataTypeStr=uint32
  M4TorqueSet_Convert : DataTypeConversion  OutDataTypeStr=uint32
  M4TorqueSet_D : Product  Inputs=*/
  M4TorqueSet_D1 : Product  Inputs=*/
  M4TorqueSet_F : Constant  Value=0.25  OutDataTypeStr=single
  M4TorqueSet_L : simulink/Logic and Bit Operations/Bitwise Operator  logicop=AND  UseBitMask=on  BitMask=65520  BitMaskRealWorld=Stored Integer
  M4TorqueSet_O : Constant  Value=-300  OutDataTypeStr=single
  M4TorqueSet_S : ArithShift  BitShiftNumber=-4
  M4TorqueSet_sat : Saturate  UpperLimit=723.75  LowerLimit=-300
  M4TorqueSet_st : Sum  Inputs=+-
  M4TorqueSetoutput6_C : Constant  Value=256
  output1 : Outport
  output2 : Outport  Port=2
  output3 : Outport  Port=3
  output4 : Outport  Port=4
  output5 : Outport  Port=5
  output6 : Outport  Port=6
  output7 : Outport  Port=7
  output8 : Outport  Port=8
  wires:
  M4TorqueSet/1 -> M4TorqueSet_sat/1
  M4TorqueSet_sat/1 -> M4TorqueSet_st/1
  M4TorqueSet_O/1 -> M4TorqueSet_st/2
  M4TorqueSet_st/1 -> M4TorqueSet_D/1
  M4TorqueSet_F/1 -> M4TorqueSet_D/2
  M4TorqueSet_D/1 -> M4TorqueSetRon/1
  M4TorqueSetRon/1 -> M4TorqueSet_S/1
  M4TorqueSet_S/1 -> M4TorqueSet_1sat/1
  M4TorqueSet_1sat/1 -> M4TorqueSet_Convert/1
  M4TorqueSet_Convert/1 -> M4TorqueSet_L/1
  M4TorqueSet_L/1 -> M4TorqueSet_D1/1, M4TorqueSet_And/1
  M4TorqueSetoutput6_C/1 -> M4TorqueSet_D1/2
  M4TorqueSet_D1/1 -> M4TorqueSetCOV/1
  M4TorqueSetCOV/1 -> output6/1
  M4TorqueSet_And_C/1 -> M4TorqueSet_And/2
  M4TorqueSet_And/1 -> M4TorqueSetBitCov/1
  M4TorqueSetBitCov/1 -> output5/1
  Constant1/1 -> output1/1
  Constant2/1 -> output2/1
  Constant3/1 -> output3/1
  Constant4/1 -> output4/1
  Constant7/1 -> output7/1
  Constant8/1 -> output8/1

== system DDCU_wxt_v02_forA_OpenLoop/OutputSignalProcess/VCU_MCU2/MCU2HeartBeat ==
  MCU2HeartBeat : Inport
  Constant{1..7} (7 alike) : Constant  Value=0  OutDataTypeStr=uint8
  MCU2HeartBeatRon : Rounding  Operator=round
  MCU2HeartBeat_1sat : Saturate  UpperLimit=240  LowerLimit=0
  MCU2HeartBeat_Convert : DataTypeConversion  OutDataTypeStr=uint8
  MCU2HeartBeat_Convert1 : DataTypeConversion  OutDataTypeStr=uint32
  MCU2HeartBeat_D : Product  Inputs=*/
  MCU2HeartBeat_F : Constant  OutDataTypeStr=single
  MCU2HeartBeat_L : simulink/Logic and Bit Operations/Bitwise Operator  logicop=AND  UseBitMask=on  BitMask=240  BitMaskRealWorld=Stored Integer
  MCU2HeartBeat_O : Constant  Value=0  OutDataTypeStr=single
  MCU2HeartBeat_S : ArithShift  BitShiftNumber=-4
  MCU2HeartBeat_sat : Saturate  UpperLimit=15  LowerLimit=0
  MCU2HeartBeat_st : Sum  Inputs=+-
  output1 : Outport
  output2 : Outport  Port=2
  output3 : Outport  Port=3
  output4 : Outport  Port=4
  output5 : Outport  Port=5
  output6 : Outport  Port=6
  output7 : Outport  Port=7
  output8 : Outport  Port=8
  wires:
  MCU2HeartBeat/1 -> MCU2HeartBeat_sat/1
  MCU2HeartBeat_sat/1 -> MCU2HeartBeat_st/1
  MCU2HeartBeat_O/1 -> MCU2HeartBeat_st/2
  MCU2HeartBeat_st/1 -> MCU2HeartBeat_D/1
  MCU2HeartBeat_F/1 -> MCU2HeartBeat_D/2
  MCU2HeartBeat_D/1 -> MCU2HeartBeatRon/1
  MCU2HeartBeatRon/1 -> MCU2HeartBeat_S/1
  MCU2HeartBeat_S/1 -> MCU2HeartBeat_1sat/1
  MCU2HeartBeat_1sat/1 -> MCU2HeartBeat_Convert1/1
  MCU2HeartBeat_Convert1/1 -> MCU2HeartBeat_L/1
  MCU2HeartBeat_L/1 -> MCU2HeartBeat_Convert/1
  MCU2HeartBeat_Convert/1 -> output8/1
  Constant1/1 -> output1/1
  Constant2/1 -> output2/1
  Constant3/1 -> output3/1
  Constant4/1 -> output4/1
  Constant5/1 -> output5/1
  Constant6/1 -> output6/1
  Constant7/1 -> output7/1

== system DDCU_wxt_v02_forA_OpenLoop/OutputSignalProcess/VCU_MCU2_replace/M3Drive ==
  M3Drive : Inport
  Constant{2..8} (7 alike) : Constant  Value=0  OutDataTypeStr=uint8
  M3DriveRon : Rounding  Operator=round
  M3Drive_1sat : Saturate  UpperLimit=48  LowerLimit=0
  M3Drive_Convert : DataTypeConversion  OutDataTypeStr=uint8
  M3Drive_Convert1 : DataTypeConversion  OutDataTypeStr=uint32
  M3Drive_D : Product  Inputs=*/
  M3Drive_F : Constant  OutDataTypeStr=single
  M3Drive_L : simulink/Logic and Bit Operations/Bitwise Operator  logicop=AND  UseBitMask=on  BitMask=48  BitMaskRealWorld=Stored Integer
  M3Drive_O : Constant  Value=0  OutDataTypeStr=single
  M3Drive_S : ArithShift  BitShiftNumber=-4
  M3Drive_sat : Saturate  UpperLimit=3  LowerLimit=0
  M3Drive_st : Sum  Inputs=+-
  output1 : Outport
  output2 : Outport  Port=2
  output3 : Outport  Port=3
  output4 : Outport  Port=4
  output5 : Outport  Port=5
  output6 : Outport  Port=6
  output7 : Outport  Port=7
  output8 : Outport  Port=8
  wires:
  M3Drive/1 -> M3Drive_sat/1
  M3Drive_sat/1 -> M3Drive_st/1
  M3Drive_O/1 -> M3Drive_st/2
  M3Drive_st/1 -> M3Drive_D/1
  M3Drive_F/1 -> M3Drive_D/2
  M3Drive_D/1 -> M3DriveRon/1
  M3DriveRon/1 -> M3Drive_S/1
  M3Drive_S/1 -> M3Drive_1sat/1
  M3Drive_1sat/1 -> M3Drive_Convert1/1
  M3Drive_Convert1/1 -> M3Drive_L/1
  M3Drive_L/1 -> M3Drive_Convert/1
  M3Drive_Convert/1 -> output1/1
  Constant2/1 -> output2/1
  Constant3/1 -> output3/1
  Constant4/1 -> output4/1
  Constant5/1 -> output5/1
  Constant6/1 -> output6/1
  Constant7/1 -> output7/1
  Constant8/1 -> output8/1

== system DDCU_wxt_v02_forA_OpenLoop/OutputSignalProcess/VCU_MCU2_replace/M3Enable ==
  M3Enable : Inport
  Constant{2..8} (7 alike) : Constant  Value=0  OutDataTypeStr=uint8
  M3EnableRon : Rounding  Operator=round
  M3Enable_1sat : Saturate  UpperLimit=3  LowerLimit=0
  M3Enable_Convert : DataTypeConversion  OutDataTypeStr=uint8
  M3Enable_Convert1 : DataTypeConversion  OutDataTypeStr=uint32
  M3Enable_D : Product  Inputs=*/
  M3Enable_F : Constant  OutDataTypeStr=single
  M3Enable_L : simulink/Logic and Bit Operations/Bitwise Operator  logicop=AND  UseBitMask=on  BitMask=3  BitMaskRealWorld=Stored Integer
  M3Enable_O : Constant  Value=0  OutDataTypeStr=single
  M3Enable_S : ArithShift
  M3Enable_sat : Saturate  UpperLimit=3  LowerLimit=0
  M3Enable_st : Sum  Inputs=+-
  output1 : Outport
  output2 : Outport  Port=2
  output3 : Outport  Port=3
  output4 : Outport  Port=4
  output5 : Outport  Port=5
  output6 : Outport  Port=6
  output7 : Outport  Port=7
  output8 : Outport  Port=8
  wires:
  M3Enable/1 -> M3Enable_sat/1
  M3Enable_sat/1 -> M3Enable_st/1
  M3Enable_O/1 -> M3Enable_st/2
  M3Enable_st/1 -> M3Enable_D/1
  M3Enable_F/1 -> M3Enable_D/2
  M3Enable_D/1 -> M3EnableRon/1
  M3EnableRon/1 -> M3Enable_S/1
  M3Enable_S/1 -> M3Enable_1sat/1
  M3Enable_1sat/1 -> M3Enable_Convert1/1
  M3Enable_Convert1/1 -> M3Enable_L/1
  M3Enable_L/1 -> M3Enable_Convert/1
  M3Enable_Convert/1 -> output1/1
  Constant2/1 -> output2/1
  Constant3/1 -> output3/1
  Constant4/1 -> output4/1
  Constant5/1 -> output5/1
  Constant6/1 -> output6/1
  Constant7/1 -> output7/1
  Constant8/1 -> output8/1

== system DDCU_wxt_v02_forA_OpenLoop/OutputSignalProcess/VCU_MCU2_replace/M3Mode ==
  M3Mode : Inport
  Constant{2..8} (7 alike) : Constant  Value=0  OutDataTypeStr=uint8
  M3ModeRon : Rounding  Operator=round
  M3Mode_1sat : Saturate  UpperLimit=12  LowerLimit=0
  M3Mode_Convert : DataTypeConversion  OutDataTypeStr=uint8
  M3Mode_Convert1 : DataTypeConversion  OutDataTypeStr=uint32
  M3Mode_D : Product  Inputs=*/
  M3Mode_F : Constant  OutDataTypeStr=single
  M3Mode_L : simulink/Logic and Bit Operations/Bitwise Operator  logicop=AND  UseBitMask=on  BitMask=12  BitMaskRealWorld=Stored Integer
  M3Mode_O : Constant  Value=0  OutDataTypeStr=single
  M3Mode_S : ArithShift  BitShiftNumber=-2
  M3Mode_sat : Saturate  UpperLimit=3  LowerLimit=0
  M3Mode_st : Sum  Inputs=+-
  output1 : Outport
  output2 : Outport  Port=2
  output3 : Outport  Port=3
  output4 : Outport  Port=4
  output5 : Outport  Port=5
  output6 : Outport  Port=6
  output7 : Outport  Port=7
  output8 : Outport  Port=8
  wires:
  M3Mode/1 -> M3Mode_sat/1
  M3Mode_sat/1 -> M3Mode_st/1
  M3Mode_O/1 -> M3Mode_st/2
  M3Mode_st/1 -> M3Mode_D/1
  M3Mode_F/1 -> M3Mode_D/2
  M3Mode_D/1 -> M3ModeRon/1
  M3ModeRon/1 -> M3Mode_S/1
  M3Mode_S/1 -> M3Mode_1sat/1
  M3Mode_1sat/1 -> M3Mode_Convert1/1
  M3Mode_Convert1/1 -> M3Mode_L/1
  M3Mode_L/1 -> M3Mode_Convert/1
  M3Mode_Convert/1 -> output1/1
  Constant2/1 -> output2/1
  Constant3/1 -> output3/1
  Constant4/1 -> output4/1
  Constant5/1 -> output5/1
  Constant6/1 -> output6/1
  Constant7/1 -> output7/1
  Constant8/1 -> output8/1

== system DDCU_wxt_v02_forA_OpenLoop/OutputSignalProcess/VCU_MCU2_replace/M3SpeedLimit ==
  M3SpeedLimit : Inport
  BitCov : DataTypeConversion  OutDataTypeStr=uint8
  Constant{1..2,5..8} (6 alike) : Constant  Value=0  OutDataTypeStr=uint8
  M3SpeedLimitCOV : DataTypeConversion  OutDataTypeStr=uint8
  M3SpeedLimitRon : Rounding  Operator=round
  M3SpeedLimit_1sat : Saturate  UpperLimit=16380  LowerLimit=0
  M3SpeedLimit_And : simulink/Logic and Bit Operations/Bitwise Operator  logicop=AND  UseBitMask=off  NumInputPorts=2  BitMask=bin2dec('11011001')  BitMaskRealWorld=Stored Integer
  M3SpeedLimit_And_C : Constant  Value=255  OutDataTypeStr=uint32
  M3SpeedLimit_Convert : DataTypeConversion  OutDataTypeStr=uint32
  M3SpeedLimit_D : Product  Inputs=*/
  M3SpeedLimit_D1 : Product  Inputs=*/
  M3SpeedLimit_F : Constant  Value=5  OutDataTypeStr=single
  M3SpeedLimit_L : simulink/Logic and Bit Operations/Bitwise Operator  logicop=AND  UseBitMask=on  BitMask=16380  BitMaskRealWorld=Stored Integer
  M3SpeedLimit_O : Constant  Value=0  OutDataTypeStr=single
  M3SpeedLimit_S : ArithShift  BitShiftNumber=-2
  M3SpeedLimit_sat : Saturate  UpperLimit=20475  LowerLimit=0
  M3SpeedLimit_st : Sum  Inputs=+-
  M3SpeedLimitoutput4_C : Constant  Value=256
  output1 : Outport
  output2 : Outport  Port=2
  output3 : Outport  Port=3
  output4 : Outport  Port=4
  output5 : Outport  Port=5
  output6 : Outport  Port=6
  output7 : Outport  Port=7
  output8 : Outport  Port=8
  wires:
  M3SpeedLimit/1 -> M3SpeedLimit_sat/1
  M3SpeedLimit_sat/1 -> M3SpeedLimit_st/1
  M3SpeedLimit_O/1 -> M3SpeedLimit_st/2
  M3SpeedLimit_st/1 -> M3SpeedLimit_D/1
  M3SpeedLimit_F/1 -> M3SpeedLimit_D/2
  M3SpeedLimit_D/1 -> M3SpeedLimitRon/1
  M3SpeedLimitRon/1 -> M3SpeedLimit_S/1
  M3SpeedLimit_S/1 -> M3SpeedLimit_1sat/1
  M3SpeedLimit_1sat/1 -> M3SpeedLimit_Convert/1
  M3SpeedLimit_Convert/1 -> M3SpeedLimit_L/1
  M3SpeedLimit_L/1 -> M3SpeedLimit_D1/1, M3SpeedLimit_And/1
  M3SpeedLimitoutput4_C/1 -> M3SpeedLimit_D1/2
  M3SpeedLimit_D1/1 -> M3SpeedLimitCOV/1
  M3SpeedLimitCOV/1 -> output4/1
  M3SpeedLimit_And_C/1 -> M3SpeedLimit_And/2
  M3SpeedLimit_And/1 -> BitCov/1
  BitCov/1 -> output3/1
  Constant1/1 -> output1/1
  Constant2/1 -> output2/1
  Constant5/1 -> output5/1
  Constant6/1 -> output6/1
  Constant7/1 -> output7/1
  Constant8/1 -> output8/1

== system DDCU_wxt_v02_forA_OpenLoop/OutputSignalProcess/VCU_MCU2_replace/M3SpeedSet ==
  M3SpeedSet : Inport
  Constant{4..8} (5 alike) : Constant  Value=0  OutDataTypeStr=uint8
  M3SpeedSetBitCov : DataTypeConversion  OutDataTypeStr=uint32
  M3SpeedSetBitCov1 : DataTypeConversion  OutDataTypeStr=uint8
  M3SpeedSetCOV : DataTypeConversion  OutDataTypeStr=uint8
  M3SpeedSetCOV1 : DataTypeConversion  OutDataTypeStr=uint8
  M3SpeedSetRon : Rounding  Operator=round
  M3SpeedSet_1sat : Saturate  UpperLimit=262080  LowerLimit=0
  M3SpeedSet_And : simulink/Logic and Bit Operations/Bitwise Operator  logicop=AND  UseBitMask=off  NumInputPorts=2  BitMask=bin2dec('11011001')  BitMaskRealWorld=Stored Integer
  M3SpeedSet_And1 : simulink/Logic and Bit Operations/Bitwise Operator  logicop=AND  UseBitMask=off  NumInputPorts=2  BitMask=bin2dec('11011001')  BitMaskRealWorld=Stored Integer
  M3SpeedSet_And1_C : Constant  Value=255  OutDataTypeStr=uint32
  M3SpeedSet_And_C : Constant  Value=65535
  M3SpeedSet_Convert : DataTypeConversion  OutDataTypeStr=uint32
  M3SpeedSet_D : Product  Inputs=*/
  M3SpeedSet_D1 : Product  Inputs=*/
  M3SpeedSet_D2 : Product  Inputs=*/
  M3SpeedSet_F : Constant  Value=5  OutDataTypeStr=single
  M3SpeedSet_L : simulink/Logic and Bit Operations/Bitwise Operator  logicop=AND  UseBitMask=on  BitMask=262080  BitMaskRealWorld=Stored Integer
  M3SpeedSet_O : Constant  Value=-5000  OutDataTypeStr=single
  M3SpeedSet_S : ArithShift  BitShiftNumber=-6
  M3SpeedSet_sat : Saturate  UpperLimit=15475  LowerLimit=-5000
  M3SpeedSet_st : Sum  Inputs=+-
  M3SpeedSetoutput2_C : Constant  Value=256
  M3SpeedSetoutput3_C : Constant  Value=65536
  output1 : Outport
  output2 : Outport  Port=2
  output3 : Outport  Port=3
  output4 : Outport  Port=4
  output5 : Outport  Port=5
  output6 : Outport  Port=6
  output7 : Outport  Port=7
  output8 : Outport  Port=8
  wires:
  M3SpeedSet/1 -> M3SpeedSet_sat/1
  M3SpeedSet_sat/1 -> M3SpeedSet_st/1
  M3SpeedSet_O/1 -> M3SpeedSet_st/2
  M3SpeedSet_st/1 -> M3SpeedSet_D/1
  M3SpeedSet_F/1 -> M3SpeedSet_D/2
  M3SpeedSet_D/1 -> M3SpeedSetRon/1
  M3SpeedSetRon/1 -> M3SpeedSet_S/1
  M3SpeedSet_S/1 -> M3SpeedSet_1sat/1
  M3SpeedSet_1sat/1 -> M3SpeedSet_Convert/1
  M3SpeedSet_Convert/1 -> M3SpeedSet_L/1
  M3SpeedSet_L/1 -> M3SpeedSet_D1/1, M3SpeedSet_And/1, M3SpeedSet_And1/1
  M3SpeedSetoutput3_C/1 -> M3SpeedSet_D1/2
  M3SpeedSet_D1/1 -> M3SpeedSetCOV/1
  M3SpeedSetCOV/1 -> output3/1
  M3SpeedSet_And_C/1 -> M3SpeedSetBitCov/1
  M3SpeedSetBitCov/1 -> M3SpeedSet_And/2
  M3SpeedSet_And/1 -> M3SpeedSet_D2/1
  M3SpeedSetoutput2_C/1 -> M3SpeedSet_D2/2
  M3SpeedSet_D2/1 -> M3SpeedSetCOV1/1
  M3SpeedSetCOV1/1 -> output2/1
  M3SpeedSet_And1_C/1 -> M3SpeedSet_And1/2
  M3SpeedSet_And1/1 -> M3SpeedSetBitCov1/1
  M3SpeedSetBitCov1/1 -> output1/1
  Constant4/1 -> output4/1
  Constant5/1 -> output5/1
  Constant6/1 -> output6/1
  Constant7/1 -> output7/1
  Constant8/1 -> output8/1

== system DDCU_wxt_v02_forA_OpenLoop/OutputSignalProcess/VCU_MCU2_replace/M4Drive ==
  M4Drive : Inport
  Constant{1..4,6..8} (7 alike) : Constant  Value=0  OutDataTypeStr=uint8
  M4DriveRon : Rounding  Operator=round
  M4Drive_1sat : Saturate  UpperLimit=12  LowerLimit=0
  M4Drive_Convert : DataTypeConversion  OutDataTypeStr=uint8
  M4Drive_Convert1 : DataTypeConversion  OutDataTypeStr=uint32
  M4Drive_D : Product  Inputs=*/
  M4Drive_F : Constant  OutDataTypeStr=single
  M4Drive_L : simulink/Logic and Bit Operations/Bitwise Operator  logicop=AND  UseBitMask=on  BitMask=12  BitMaskRealWorld=Stored Integer
  M4Drive_O : Constant  Value=0  OutDataTypeStr=single
  M4Drive_S : ArithShift  BitShiftNumber=-2
  M4Drive_sat : Saturate  UpperLimit=3  LowerLimit=0
  M4Drive_st : Sum  Inputs=+-
  output1 : Outport
  output2 : Outport  Port=2
  output3 : Outport  Port=3
  output4 : Outport  Port=4
  output5 : Outport  Port=5
  output6 : Outport  Port=6
  output7 : Outport  Port=7
  output8 : Outport  Port=8
  wires:
  M4Drive/1 -> M4Drive_sat/1
  M4Drive_sat/1 -> M4Drive_st/1
  M4Drive_O/1 -> M4Drive_st/2
  M4Drive_st/1 -> M4Drive_D/1
  M4Drive_F/1 -> M4Drive_D/2
  M4Drive_D/1 -> M4DriveRon/1
  M4DriveRon/1 -> M4Drive_S/1
  M4Drive_S/1 -> M4Drive_1sat/1
  M4Drive_1sat/1 -> M4Drive_Convert1/1
  M4Drive_Convert1/1 -> M4Drive_L/1
  M4Drive_L/1 -> M4Drive_Convert/1
  M4Drive_Convert/1 -> output5/1
  Constant1/1 -> output1/1
  Constant2/1 -> output2/1
  Constant3/1 -> output3/1
  Constant4/1 -> output4/1
  Constant6/1 -> output6/1
  Constant7/1 -> output7/1
  Constant8/1 -> output8/1

== system DDCU_wxt_v02_forA_OpenLoop/OutputSignalProcess/VCU_MCU2_replace/M4Enable ==
  M4Enable : Inport
  Constant{1..3,5..8} (7 alike) : Constant  Value=0  OutDataTypeStr=uint8
  M4EnableRon : Rounding  Operator=round
  M4Enable_1sat : Saturate  UpperLimit=192  LowerLimit=0
  M4Enable_Convert : DataTypeConversion  OutDataTypeStr=uint8
  M4Enable_Convert1 : DataTypeConversion  OutDataTypeStr=uint32
  M4Enable_D : Product  Inputs=*/
  M4Enable_F : Constant  OutDataTypeStr=single
  M4Enable_L : simulink/Logic and Bit Operations/Bitwise Operator  logicop=AND  UseBitMask=on  BitMask=192  BitMaskRealWorld=Stored Integer
  M4Enable_O : Constant  Value=0  OutDataTypeStr=single
  M4Enable_S : ArithShift  BitShiftNumber=-6
  M4Enable_sat : Saturate  UpperLimit=3  LowerLimit=0
  M4Enable_st : Sum  Inputs=+-
  output1 : Outport
  output2 : Outport  Port=2
  output3 : Outport  Port=3
  output4 : Outport  Port=4
  output5 : Outport  Port=5
  output6 : Outport  Port=6
  output7 : Outport  Port=7
  output8 : Outport  Port=8
  wires:
  M4Enable/1 -> M4Enable_sat/1
  M4Enable_sat/1 -> M4Enable_st/1
  M4Enable_O/1 -> M4Enable_st/2
  M4Enable_st/1 -> M4Enable_D/1
  M4Enable_F/1 -> M4Enable_D/2
  M4Enable_D/1 -> M4EnableRon/1
  M4EnableRon/1 -> M4Enable_S/1
  M4Enable_S/1 -> M4Enable_1sat/1
  M4Enable_1sat/1 -> M4Enable_Convert1/1
  M4Enable_Convert1/1 -> M4Enable_L/1
  M4Enable_L/1 -> M4Enable_Convert/1
  M4Enable_Convert/1 -> output4/1
  Constant1/1 -> output1/1
  Constant2/1 -> output2/1
  Constant3/1 -> output3/1
  Constant5/1 -> output5/1
  Constant6/1 -> output6/1
  Constant7/1 -> output7/1
  Constant8/1 -> output8/1
